simulink model "sim2"  (R2023b)
settings: Solver=VariableStepAuto  StartTime=0.0  StopTime=10.0  RelTol=1e-3
values from neighbouring files (symbols this model uses):
  Kiid = 1    [sim1_variables.m]
  Kiiq = 1    [sim1_variables.m]
  Kivel = 1    [sim1_variables.m]
  Kpid = 1    [sim1_variables.m]
  Kpiq = 1    [sim1_variables.m]
  Kpvel = 1    [sim1_variables.m]
  Tsw = 1/100    (= 0.01)    [sim1_variables.m]
undefined symbols (not defined in the file or in its folder): N
libraries: nesl_utility x14, fl_lib x9, ee_lib x9, eeTransforms x3, slpidlib x3, simulink x2, batteryecm_lib x1, simulink_extras x1, eePwmGeneratorTwoLevel x1
(part 2 of 2)

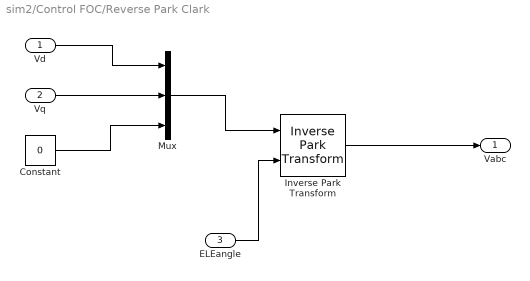
== system sim2/Control FOC/Reverse Park Clark ==
  Vd : Inport
  Vq : Inport  Port=2
  ELEangle : Inport  Port=3
  Constant : Constant  Value=0
  Inverse Park Transform : eeTransforms/Inverse Park Transform  AxisAlignment=Q-axis  PowerInvariant=off
      settings: LibrarySourceBlock=|
      | ee_sl_lib/Mathematical
      | Transforms/Inverse
      | Park Transform
  Mux : Mux  Inputs=3
  Vabc : Outport
  wires:
  Vd/1 -> Mux/1
  Vq/1 -> Mux/2
  Constant/1 -> Mux/3
  Mux/1 -> Inverse Park Transform/1
  ELEangle/1 -> Inverse Park Transform/2
  Inverse Park Transform/1 -> Vabc/1

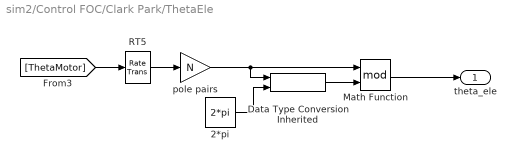
== system sim2/Control FOC/Clark Park/ThetaEle ==
  2*pi : Constant  Value=2*pi  OutDataTypeStr=Inherit: Inherit via back propagation  SampleTime=2e-4
  Data Type Conversion Inherited : simulink/Signal Attributes/Data Type Conversion Inherited  ConvertRealWorld=Real World Value  DoSatur=off
  Math Function : Math  Operator=mod  SignedPower=on
  RT5 : RateTransition  OutPortSampleTime=Tspeed
  "pole pairs " : Gain  Gain=N
  theta_ele : Outport  VectorParamsAs1DForOutWhenUnconnected=off
  wires:
  [ThetaMotor] -> RT5/1
  Math Function/1 -> theta_ele/1
  RT5/1 -> "pole pairs "/1
  2*pi/1 -> Data Type Conversion Inherited/2
  "pole pairs "/1 -> Data Type Conversion Inherited/1, Math Function/1
  Data Type Conversion Inherited/1 -> Math Function/2

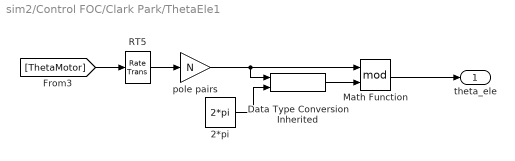
== system sim2/Control FOC/Clark Park/ThetaEle1 ==
  2*pi : Constant  Value=2*pi  OutDataTypeStr=Inherit: Inherit via back propagation  SampleTime=2e-4
  Data Type Conversion Inherited : simulink/Signal Attributes/Data Type Conversion Inherited  ConvertRealWorld=Real World Value  DoSatur=off
  Math Function : Math  Operator=mod  SignedPower=on
  RT5 : RateTransition  OutPortSampleTime=Tspeed
  "pole pairs " : Gain  Gain=N
  theta_ele : Outport  VectorParamsAs1DForOutWhenUnconnected=off
  wires:
  Data Type Conversion Inherited/1 -> Math Function/2
  "pole pairs "/1 -> Math Function/1, Data Type Conversion Inherited/1
  2*pi/1 -> Data Type Conversion Inherited/2
  RT5/1 -> "pole pairs "/1
  Math Function/1 -> theta_ele/1
  [ThetaMotor] -> RT5/1
